simulink model "regulkatorPID"  (R2021b)
settings: Solver=VariableStepAuto  StartTime=0.0  StopTime=300  RelTol=1e-3
settings Model: Creator=mateusznowak  LastModifiedBy=mateusznowak

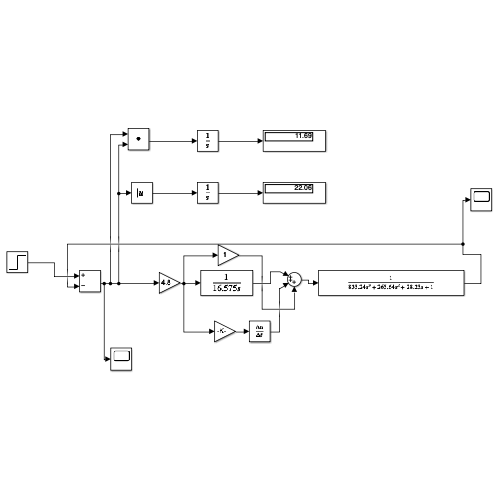
[thumbnail: Simulink's stored preview of the top-level diagram]
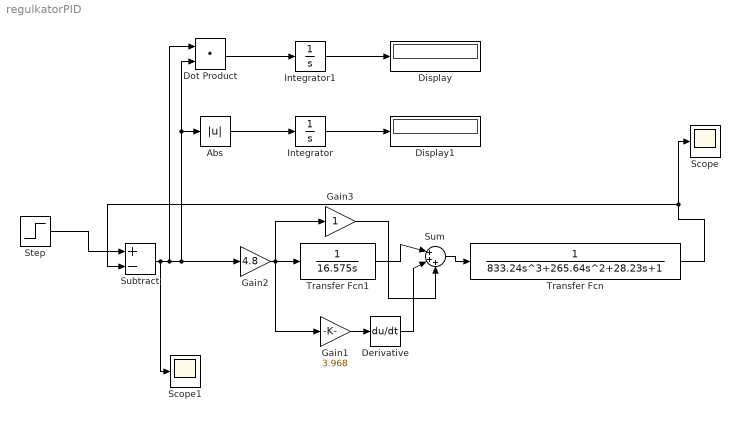
== system regulkatorPID ==
  Abs : Abs
  Derivative : Derivative
  Display : Display
  Display1 : Display
  Dot Product : DotProduct  InputSameDT=on  OutDataTypeStr=Inherit: Inherit via internal rule
  Gain1 : Gain  Gain=3.968
  Gain2 : Gain  Gain=4.8
  Gain3 : Gain
  Integrator : Integrator
  Integrator1 : Integrator
  Scope : Scope
  Scope1 : Scope
  Step : Step  SampleTime=0
  Subtract : Sum  Inputs=+-
  Sum : Sum  Inputs=|+++
  Transfer Fcn : TransferFcn  Denominator=[833.24 265.64 28.23 1]
  Transfer Fcn1 : TransferFcn  Denominator=[16.575 0]
  wires:
  Transfer Fcn1/1 -> Sum/1
  Integrator/1 -> Display1/1
  Dot Product/1 -> Integrator1/1
  Subtract/1 -> Scope1/1, Dot Product/1, Gain2/1, Dot Product/2, Abs/1
  Sum/1 -> Transfer Fcn/1
  Step/1 -> Subtract/1
  Gain2/1 -> Gain3/1, Gain1/1, Transfer Fcn1/1
  Abs/1 -> Integrator/1
  Transfer Fcn/1 -> Scope/1, Subtract/2
  Integrator1/1 -> Display/1
  Gain1/1 -> Derivative/1
  Derivative/1 -> Sum/2
  Gain3/1 -> Sum/3
